simulink model "testsplitter"  (R2012b)
settings: Solver=ode45  StartTime=0.0  StopTime=10.0  RelTol=1e-3
settings Model: Creator=tlavelle  LastModifiedBy=tlavelle

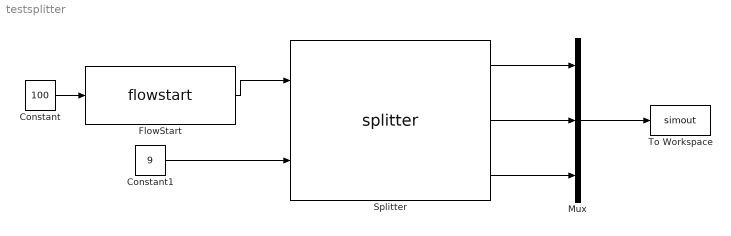
== system testsplitter ==
  Constant : Constant  Value=100
  Constant1 : Constant  Value=9
  FlowStart : M-S-Function  FunctionName=flowstart  Parameters=Tt,Pt,comp1,comp2,comp3,comp4,comp5,comp6  mask{Tt=500, Pt=15, comp1=1, comp2=0, comp3=0, comp4=0, comp5=0, comp6=0}
      mask prompts: Tt "Exit Temperature"; Pt "Exit Pressure"
      mask Display:
      | color('red'); port_label('input',1,'Flow')
      | color('red'); port_label('output',1,'Flow Out')
  Mux : Mux  Inputs=3
  "Splitter " : M-S-Function  FunctionName=splitter
      mask Display:
      | color('red'); port_label('input',1,'Flow In')
      | color('red'); port_label('input',2,'BPR')
      | 
      | color('red'); port_label('output',1,'Flow Secondary')
      | color('red'); port_label('output',2,'Flow Primary')
  To Workspace : ToWorkspace  VariableName=simout  SampleTime=-1  SaveFormat=Timeseries
  wires:
  Constant/1 -> FlowStart/1
  FlowStart/1 -> "Splitter "/1
  Constant1/1 -> "Splitter "/2
  "Splitter "/1 -> Mux/1
  "Splitter "/2 -> Mux/2
  Mux/1 -> To Workspace/1
  "Splitter "/3 -> Mux/3
